simulink model "MEMS_Gyro_SenseModeControl"  (R2022b)
settings: Solver=VariableStepAuto  StartTime=0.0  StopTime=10  MaxStep=1e-5  RelTol=1e-3
libraries: dsparch4 x1, slpidlib x1
settings Model: Creator=Rio  LastModifiedBy=Rio

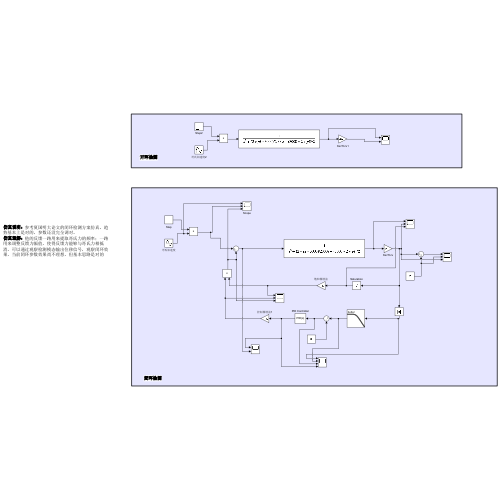
[thumbnail: Simulink's stored preview of the top-level diagram]
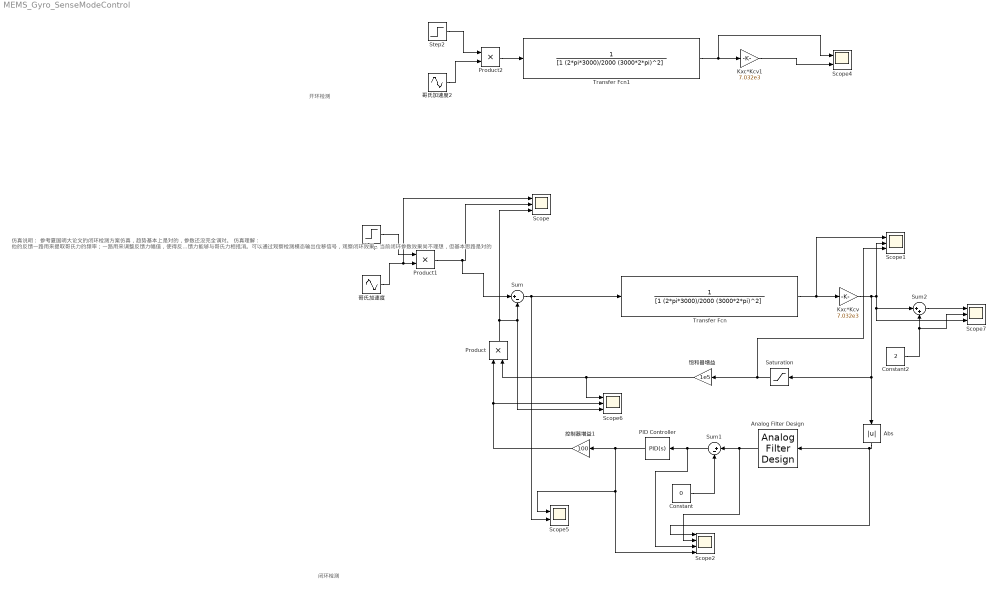
== system MEMS_Gyro_SenseModeControl ==
  note: 闭环检测
  note: 仿真说明： 参考夏国明大论文的闭环检测方案仿真，趋势基本上是对的，参数还没完全调对。
      | 仿真理解： 他的反馈一路用来提取哥氏力的频率；一路用来调整反馈力幅值，使得反馈力能够与哥氏力相抵消。可以通过观察检测模态输出位移信号，观察闭环效果，当前闭环参数效果尚不理想，但基本思路是对的
  note: 开环检测
  Abs : Abs  SaturateOnIntegerOverflow=off
  Analog Filter Design : dsparch4/Analog Filter Design  method=Butterworth  filttype=Lowpass  N=2  Wlo=2*pi*100  Whi=80  Rp=2  Rs=40
  Constant : Constant  Value=0
  Constant2 : Constant  Value=2
  Kxc*Kcv : Gain  Gain=7.032e3
  Kxc*Kcv1 : Gain  Gain=7.032e3
  PID Controller : slpidlib/PID Controller  Controller=PID  Form=Parallel  TimeDomain=Continuous-time  UseExternalTs=off  SampleTime=-1  IntegratorMethod=Forward Euler  FilterMethod=Forward Euler  ControllerParametersSource=internal  P=50  I=30  UseKiTs=off  D=0  N=100  UseFilter=on  TunerSelectOption=Transfer Function Based (PID Tuner App)  InitialConditionSource=internal  InitialConditionForIntegrator=0  InitialConditionForFilter=0  DifferentiatorICPrevScaledInput=0  ExternalReset=none  TrackingMode=off  Kt=1  LimitOutput=off  SatLimitsSource=internal  UpperSaturationLimit=inf  LowerSaturationLimit=-inf  LinearizeAsGain=on  AntiWindupMode=none  Kb=1  LimitIntegrator=off  UpperIntegratorSaturationLimit=inf  LowerIntegratorSaturationLimit=-inf  POutMin=[]  POutMax=[]  IOutMin=[]  IOutMax=[]  DOutMin=[]  DOutMax=[]  NOutMin=[]  NOutMax=[]  SumOutMin=[]  SumOutMax=[]  SaturationOutMin=[]  SaturationOutMax=[]  PParamMin=[]  PParamMax=[]  IParamMin=[]  IParamMax=[]  DParamMin=[]  DParamMax=[]  NParamMin=[]  NParamMax=[]  KbParamMin=[]  KbParamMax=[]  KtParamMin=[]  KtParamMax=[]  KbOutMin=[]  KbOutMax=[]  KtOutMin=[]  KtOutMax=[]  IntegratorOutMin=[]  IntegratorOutMax=[]  FilterOutMin=[]  FilterOutMax=[]  SumI1OutMin=[]  SumI1OutMax=[]  SumI2OutMin=[]  SumI2OutMax=[]  SumI3OutMin=[]  SumI3OutMax=[]  SumI4OutMin=[]  SumI4OutMax=[]  SumDOutMin=[]  SumDOutMax=[]  DifferentiatorOutMin=[]  DifferentiatorOutMax=[]  FilterDiffOutCoefMin=[]  FilterDiffOutCoefMax=[]  ReciprocalOutMin=[]  ReciprocalOutMax=[]  SumDenOutMin=[]  SumDenOutMax=[]  SumNumOutMin=[]  SumNumOutMax=[]  DivideOutMin=[]  DivideOutMax=[]  UdiffTsProdOutMin=[]  UdiffTsProdOutMax=[]  NTsProdOutMin=[]  NTsProdOutMax=[]  UintegralTsProdOutMin=[]  UintegralTsProdOutMax=[]  UngainTsProdOutMin=[]  UngainTsProdOutMax=[]  ClampingZeroOutDataTypeStr=Inherit: Inherit via back propagation  ClampingZeroOutMin=[]  ClampingZeroOutMax=[]  FilterDenConstantOutDataTypeStr=Inherit: Inherit via back propagation  FilterDenConstantOutMin=[]  FilterDenConstantOutMax=[]  PCopyOutDataTypeStr=Inherit: Inherit via back propagation  PCopyOutMin=[]  PCopyOutMax=[]  NCopyOutDataTypeStr=Inherit: Inherit via back propagation  NCopyOutMin=[]  NCopyOutMax=[]  IntegratorContinuousStateAttributes=''  IntegratorStateMustResolveToSignalObject=off  IntegratorRTWStateStorageClass=Auto  FilterContinuousStateAttributes=''  FilterStateMustResolveToSignalObject=off  FilterRTWStateStorageClass=Auto  ParallelPVariant=InternalParameters  IdealPVariant=Disabled  IVariant=InternalParameters  DVariant=InternalParameters  IntegratorVariant=Continuous  SatVariant=Disabled  AWVariant=Passthrough  PCopyVariant=Disabled  TRVariant=Disabled  FdbkBlocksVariant=Forward  IdealPFdbkVariant=Disabled  SatFdbkVariant=Disabled  DerivativeFilterVariant=ContFilter  NVariant=InternalParameters  NCopyVariant=Disabled  FilterICVariant=InternalICsFilter  IntegratorICVariant=InternalICs  ExternalResetVariant=Disabled  TRSumVariant=Passthrough  SumFdbkVariant=Disabled  SumVariant=Sum_PID  TsampFilterVariant=InternalTs  TsampNgainVariant=Passthrough  TsampIntegralVariant=Passthrough  ExternalSaturationOutDataTypeStr=Inherit: Same as second input
  Product : Product
  Product1 : Product
  Product2 : Product
  Saturation : Saturate  UpperLimit=1e-5  LowerLimit=-1e-5
  Scope{,1,6..7} (4 alike) : Scope  NumInputPorts=3
  Scope2 : Scope  NumInputPorts=4
  Scope4 : Scope  NumInputPorts=2
  Scope5 : Scope  NumInputPorts=2
  Step : Step  Time=0.5  SampleTime=0
  Step2 : Step  Time=0.5  SampleTime=0
  Sum : Sum  Inputs=|+-
  Sum1 : Sum  Inputs=|+-
  Sum2 : Sum  Inputs=|++
  Transfer Fcn : TransferFcn  Denominator=[1 (2*pi*3000)/2000 (3000*2*pi)^2]
  Transfer Fcn1 : TransferFcn  Denominator=[1 (2*pi*3000)/2000 (3000*2*pi)^2]
  哥氏加速度 : Sin  Frequency=2*pi*2900  SampleTime=0
  哥氏加速度2 : Sin  Frequency=2*pi*2900  SampleTime=0
  控制器增益1 : Gain  Gain=100
  饱和器增益 : Gain  Gain=1e5
  wires:
  Transfer Fcn/1 -> Scope1/1, Kxc*Kcv/1
  Kxc*Kcv/1 -> Scope7/3, Sum2/1, Scope1/2, Abs/1, Saturation/1
  Abs/1 -> Scope2/1, Analog Filter Design/1
  PID Controller/1 -> Scope5/1, Scope2/4, 控制器增益1/1
  Saturation/1 -> Scope1/3, 饱和器增益/1
  Analog Filter Design/1 -> Scope2/2, Sum1/1
  Sum1/1 -> Scope2/3, PID Controller/1
  Constant/1 -> Sum1/2
  Step/1 -> Product1/1
  哥氏加速度/1 -> Scope/1, Product1/2
  Product1/1 -> Sum/1, Scope/2
  Product2/1 -> Transfer Fcn1/1
  Transfer Fcn1/1 -> Scope4/1, Kxc*Kcv1/1
  哥氏加速度2/1 -> Product2/2
  Step2/1 -> Product2/1
  Kxc*Kcv1/1 -> Scope4/2
  饱和器增益/1 -> Scope6/1, Product/2
  控制器增益1/1 -> Product/1, Scope6/2
  Product/1 -> Scope/3, Scope6/3, Sum/2
  Sum/1 -> Transfer Fcn/1, Scope5/2
  Constant2/1 -> Scope7/2, Sum2/2
  Sum2/1 -> Scope7/1
